simulink model "Orbit_Propagator"  (R2020b)
settings: Solver=FixedStepAuto  StartTime=0.0  StopTime=50000  FixedStep=1  RelTol=1e-5
PostLoadFcn:
  | if builtin('license','test','Virtual_Reality_Toolbox')
  |     set_param([bdroot(gcs) '/Simulink 3D Animation'], 'enableVis', 'on')
  | else
  |     set_param([bdroot(gcs) '/Simulink 3D Animation'], 'enableVis', 'off')
  | end
InitFcn:
  | if strcmp(get_param([bdroot(gcs) '/Simulink 3D Animation'], 'enableVis'), 'on')
  |     if ~builtin('license','checkout','Virtual_Reality_Toolbox')
  |         error(message('aeroblks_cubesat:cubesat:licenseFailAnimTemplate'));
  |     end
  | end
model workspace (MATLAB code in the model file + MAT data in the model file):
  aeroCoeff : object (value not decoded)
  environment : EarthRefAlt (value not decoded)
  initCond : object (value not decoded)
  inputs0 : object (value not decoded)
  states0 : object (value not decoded)
  vehicle : object (value not decoded)
  other statements: initialize6DOFSkyHogg;
undefined symbols (not defined in the file): constraintAxes, deg, Earth, euler0, juliandate, km, pointing, pqr0, rad, s, WGS84, WMM2020
libraries: aerolibutil x11, aerolibconvert2 x7, sharedtransform x3, aerolibattitudesys x2, aerolibcelestial x2, simulink x2, aerolibgravity2 x2, aerolibcubesat x1, aerolib6dof2 x1, pid_lib x1, aerolibobsolete x1, vrlib x1
(part 2 of 2)

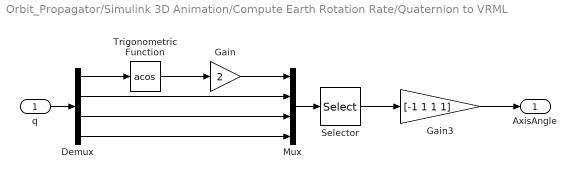
== system Orbit_Propagator/Simulink 3D Animation/Compute Earth Rotation Rate/Quaternion to VRML ==
  q : Inport
  Demux : Demux
  Gain : Gain  Gain=2
  Gain3 : Gain  Gain=[-1 1 1 1]
  Mux : Mux
  Selector : Selector  InputPortWidth=4  IndexOptions=Index vector (dialog)  Indices=[2 4 3 1]  OutputSizes=1
  Trigonometric Function : Trigonometry  Operator=acos
  AxisAngle : Outport  VectorParamsAs1DForOutWhenUnconnected=off
  wires:
  Demux/1 -> Trigonometric Function/1
  Trigonometric Function/1 -> Gain/1
  Mux/1 -> Selector/1
  q/1 -> Demux/1
  Gain3/1 -> AxisAngle/1
  Selector/1 -> Gain3/1
  Gain/1 -> Mux/1
  Demux/2 -> Mux/2
  Demux/3 -> Mux/3
  Demux/4 -> Mux/4

== system Orbit_Propagator/Simulink 3D Animation/Compute Umbra Translation/unitVec ==
  I : Inport
  Divide : Product  Inputs=*/
  Dot Product : DotProduct  InputSameDT=on  OutDataTypeStr=Inherit: Inherit via internal rule
  Sqrt : Sqrt  SaturateOnIntegerOverflow=on
  O : Outport  VectorParamsAs1DForOutWhenUnconnected=off
  wires:
  Dot Product/1 -> Sqrt/1
  I/1 -> Divide/1, Dot Product/1, Dot Product/2
  Divide/1 -> O/1
  Sqrt/1 -> Divide/2

== system Orbit_Propagator/Simulink 3D Animation/Sat Position to VRML/ECEF to VRML ==
  M : Inport  PortDimensions=3
  Selector : Selector  InputPortWidth=3  IndexOptions=Index vector (dialog)  Indices=[2 3 1]  OutputSizes=1
  VR : Outport  PortDimensions=3  VectorParamsAs1DForOutWhenUnconnected=off
  wires:
  M/1 -> Selector/1
  Selector/1 -> VR/1

== system Orbit_Propagator/Simulink 3D Animation/Sun Position to VRML/ECEF to VRML ==
  M : Inport  PortDimensions=3
  Selector : Selector  InputPortWidth=3  IndexOptions=Index vector (dialog)  Indices=[2 3 1]  OutputSizes=1
  VR : Outport  PortDimensions=3  VectorParamsAs1DForOutWhenUnconnected=off
  wires:
  M/1 -> Selector/1
  Selector/1 -> VR/1

== matlab function Orbit_Propagator/MATLAB Function3 ==
  data: jd input; dyear output
function dyear = jd2dyear(jd)

dyear = ((jd-2458849.5)/365.25)+2020;
end

== matlab function Orbit_Propagator/MATLAB Function4 ==
  data: x input; v output; y input; z input
function v = fcn(x, y, z)

v = sqrt(x^2 + y^2 + z^2);
end

== matlab function Orbit_Propagator/MATLAB Function9 ==
  data: cameraDir input; pullmanDir input; theta output
function theta = fcn(cameraDir, pullmanDir)
% #codegen
x = dot(cameraDir, pullmanDir) / (norm(cameraDir)*norm(pullmanDir));

theta = acos(x);

== matlab function Orbit_Propagator/MATLAB Function1 ==
  data: x input; v output; y input; z input
function v = fcn(x, y, z)

v = sqrt(x^2 + y^2 + z^2);
end
